simulink model "Model_double_control"  (R2019b)
settings: Solver=FixedStepAuto  StartTime=0.0  StopTime=0.1  RelTol=1e-3
values from neighbouring files (symbols this model uses):
  c = 14.86e-12    (= 1.486e-11)    [Q_fac.m]
  frequency = 13.56e6    (= 13560000)    [Q_fac.m]
  k_mrc = 1/q    [Q_fac.m]
  r = 50    [Q_fac.m]
libraries: simulink x10, nesl_utility x9, ee_lib x7, fl_lib x7, dspstat3 x4, powerlib_meascontrol x4
settings Model: Creator=Kia  LastModifiedBy=Kia

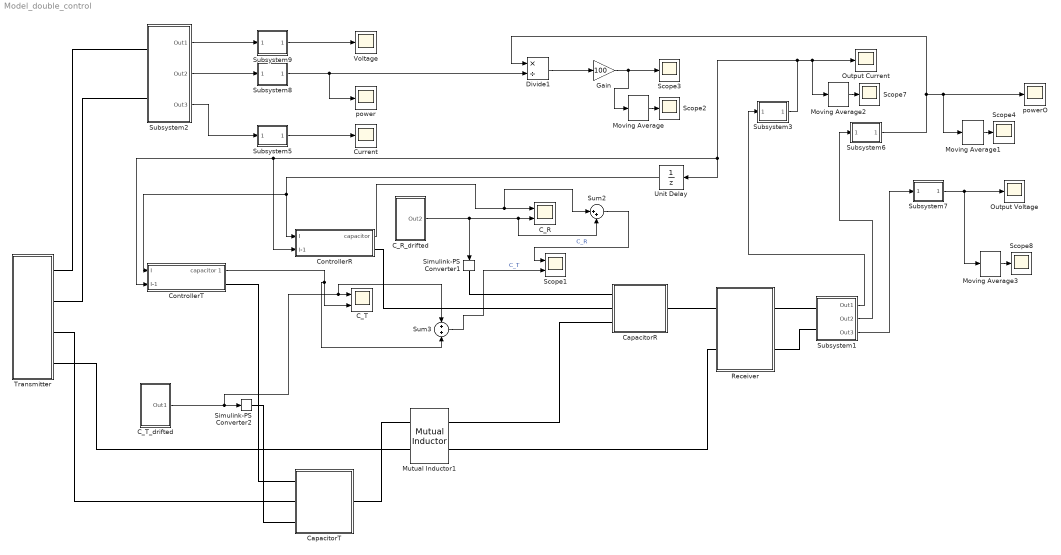
== system Model_double_control ==
  C_R : Scope  NumInputPorts=2
  C_R_drifted : Subsystem
  C_T : Scope  NumInputPorts=2
  C_T_drifted : Subsystem
  CapacitorR : Subsystem
  CapacitorT : Subsystem
  ControllerR : Subsystem
  ControllerT : Subsystem
  Current : Scope
  Divide1 : Product  Inputs=*/
  Gain : Gain  Gain=100
  Moving Average{,1..3} (4 alike) : dspstat3/Moving Average  Method=Sliding window  ForgettingFactorPort=off  SpecifyWindowLength=on  WindowLength=10  ForgettingFactor=0.9  SimulateUsing=Code generation
  Mutual Inductor1 : fl_lib/Electrical/Electrical Elements/Mutual Inductor  L1=l H  L2=l H  k=k_mrc  i1_specify=off  i1_priority=High  i1=0 A  i1_nominal_specify=off  i1_nominal_unit=A  i1_nominal_value=1  i2_specify=off  i2_priority=High  i2=0 A  i2_nominal_specify=off  i2_nominal_unit=A  i2_nominal_value=1  v1_specify=off  v1_priority=None  v1=0 V  v1_nominal_specify=off  v1_nominal_unit=V  v1_nominal_value=1  v2_specify=off  v2_priority=None  v2=0 V  v2_nominal_specify=off  v2_nominal_unit=V  v2_nominal_value=1
      settings: SourceProductName=Simscape  SourceProductBaseCode=SS  InternalSimscapePortConfiguration="{\"Bottom\":[],\"Left\":[{\"id\":\"p1\",\"label\":\"1+\",\"type\":\"foundation.electrical.electrical\"},{\"id\":\"n1\",\"label\":\"1-\",\"type\":\"foundation.electrical.electrical\"}],\"Right\":[{\"id\":\"p2\",\"label\":\"2+\",\"type\":\"foundation.electrical.electrical\"},{\"id\":\"n2\",\"label\":\"2-\",\"type\":\"foundation.electrical.electrical\"}],\"Top\":[]}"
  Output Current : Scope
  Output Voltage : Scope
  Receiver : Subsystem
  Scope1 : Scope  NumInputPorts=2
  Scope{2..4,7..8} (5 alike) : Scope
  Simulink-PS Converter1 : nesl_utility/Simulink-PS Converter  PhysicalDomain=network_engine_domain  SubClassName=ps_input  LeftPortType=input  RightPortType=output  PseudoPeriodic=off  Frequencies=[]  NoiseDistribution=none  NoiseParameters=[]  Unit=1  AffineConversion=off  FilteringAndDerivatives=provide  SimscapeFilterOrder=1  InputFilterTimeConstant=0.001  UdotUserProvided=0
  Simulink-PS Converter2 : nesl_utility/Simulink-PS Converter  PhysicalDomain=network_engine_domain  SubClassName=ps_input  LeftPortType=input  RightPortType=output  PseudoPeriodic=off  Frequencies=[]  NoiseDistribution=none  NoiseParameters=[]  Unit=1  AffineConversion=off  FilteringAndDerivatives=provide  SimscapeFilterOrder=1  InputFilterTimeConstant=0.001  UdotUserProvided=0
  Subsystem1 : Subsystem
  Subsystem2 : Subsystem
  Subsystem3 : Subsystem
  Subsystem5 : Subsystem
  Subsystem6 : Subsystem
  Subsystem7 : Subsystem
  Subsystem8 : Subsystem
  Subsystem9 : Subsystem
  Sum2 : Sum  Inputs=|++
  Sum3 : Sum  Inputs=+|+
  Transmitter : Subsystem
  Unit Delay : UnitDelay  SampleTime=2e-5  HasFrameUpgradeWarning=on
  Voltage : Scope
  power : Scope
  powerO : Scope
  wires:
  Subsystem1/3(Out3) -> Subsystem7/1(In1)
  Subsystem2/3(Out3) -> Subsystem5/1(In1)
  Subsystem1/2(Out2) -> Subsystem6/1(In1)
  Subsystem2/2(Out2) -> Subsystem8/1(In1)
  Subsystem2/1(Out1) -> Subsystem9/1(In1)
  Subsystem1/1(Out1) -> Subsystem3/1(In1)
  ControllerR/1("capacitor ") -> Sum2/1, C_R/1
  Subsystem3/1(Out1) -> Moving Average2/1, Output Current/1, Unit Delay/1, ControllerR/2(I-1), ControllerT/2(I-1)
  Subsystem6/1(Out1) -> Moving Average1/1, powerO/1, Divide1/1
  Divide1/1 -> Gain/1
  C_R_drifted/1(Out2) -> Sum2/2, C_R/2, Simulink-PS Converter1/1
  C_T_drifted/1(Out1) -> Sum3/1, C_T/1, Simulink-PS Converter2/1
  Sum2/1 -> Scope1/1  "C_R"
  Sum3/1 -> Scope1/2  "C_T"
  Unit Delay/1 -> ControllerT/1(I), ControllerR/1(I)
  Subsystem7/1(Out1) -> Moving Average3/1, Output Voltage/1
  Subsystem8/1(Out1) -> power/1, Divide1/2
  Subsystem5/1(Out1) -> Current/1
  Subsystem9/1(Out1) -> Voltage/1
  Gain/1 -> Moving Average/1, Scope3/1
  Moving Average/1 -> Scope2/1
  Moving Average1/1 -> Scope4/1
  Moving Average2/1 -> Scope7/1
  Moving Average3/1 -> Scope8/1
  ControllerT/1(capacitor 1) -> C_T/2, Sum3/2
  connections:
  Receiver/RConn2 -- Subsystem1/LConn2
  Transmitter/RConn3 -- CapacitorT/LConn2
  Transmitter/RConn2 -- Subsystem2/LConn2
  Simulink-PS Converter1/RConn1 -- CapacitorR/LConn1
  Receiver/RConn1 -- Subsystem1/LConn1
  Transmitter/RConn1 -- Subsystem2/LConn1
  Mutual Inductor1/LConn2 -- Transmitter/RConn4
  Mutual Inductor1/RConn2 -- Receiver/LConn2
  Receiver/LConn1 -- CapacitorR/RConn1
  CapacitorR/LConn3 -- Mutual Inductor1/RConn1
  ControllerR/RConn1 -- CapacitorR/LConn2
  CapacitorT/RConn1 -- Mutual Inductor1/LConn1
  Simulink-PS Converter2/RConn1 -- CapacitorT/LConn3
  ControllerT/RConn1 -- CapacitorT/LConn1

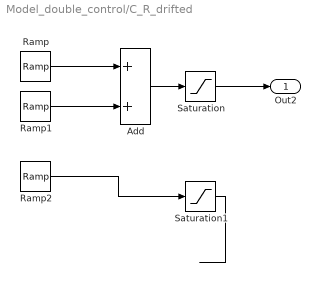
== system Model_double_control/C_R_drifted ==
  Add : Sum
  Ramp : simulink/Sources/Ramp  slope=(0.05*c)*1/2e-4  start=0.015  InitialOutput=0.5*c
  Ramp1 : simulink/Sources/Ramp  slope=-(0.05*c)*2/2e-4  start=0.019  InitialOutput=0
  Ramp2 : simulink/Sources/Ramp  slope=(0.05*c)*1/10e-3  start=0.03  InitialOutput=0.5*c
  Saturation : Saturate  UpperLimit=0.55*c  LowerLimit=c/2
  Saturation1 : Saturate  UpperLimit=0.55*c  LowerLimit=c/2
  Out2 : Outport
  wires:
  Ramp/1 -> Add/1
  Ramp1/1 -> Add/2
  Add/1 -> Saturation/1
  Saturation/1 -> Out2/1
  Saturation1/1 -> ?
  Ramp2/1 -> Saturation1/1

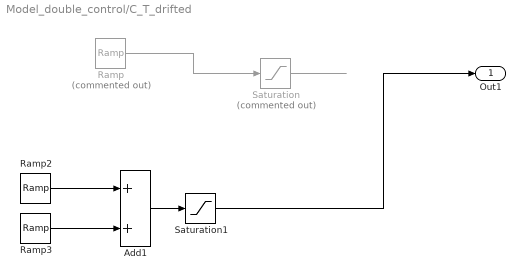
== system Model_double_control/C_T_drifted ==
  Add1 : Sum
  Ramp : simulink/Sources/Ramp  Commented=on  slope=(0.05*c)*1/10e-3  start=1e-4  InitialOutput=0.5*c
  Ramp2 : simulink/Sources/Ramp  slope=(0.05*c)*1/2e-4  start=1e-4  InitialOutput=0.5*c
  Ramp3 : simulink/Sources/Ramp  slope=-(0.05*c)*2/2e-4  start=0.004  InitialOutput=0
  Saturation : Saturate  Commented=on  UpperLimit=0.55*c  LowerLimit=c/2
  Saturation1 : Saturate  UpperLimit=0.55*c  LowerLimit=c/2
  Out1 : Outport
  wires:
  Ramp/1 -> Saturation/1
  Saturation/1 -> ?
  Ramp3/1 -> Add1/2
  Add1/1 -> Saturation1/1
  Ramp2/1 -> Add1/1
  Saturation1/1 -> Out1/1

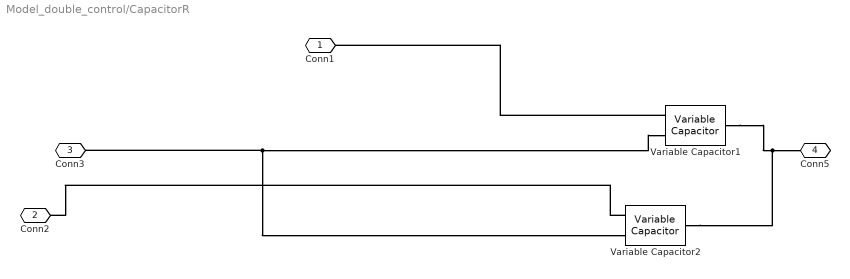
== system Model_double_control/CapacitorR ==
  Variable Capacitor1 : ee_lib/Passive/Variable Capacitor  prm=2  Cmin=1e-20 F  r=0 Ohm  v0=0 V  q0=0 C
      settings: SourceProductName=Simscape Electrical  SourceProductBaseCode=PS  InternalSimscapePortConfiguration="{\"Bottom\":[],\"Left\":[{\"id\":\"C\",\"label\":\"C\",\"type\":\"input\"},{\"id\":\"p\",\"label\":\"+\",\"type\":\"foundation.electrical.electrical\"}],\"Right\":[{\"id\":\"n\",\"label\":\"-\",\"type\":\"foundation.electrical.electrical\"}],\"Top\":[]}"
  Variable Capacitor2 : ee_lib/Passive/Variable Capacitor  prm=2  Cmin=1e-20 F  r=0 Ohm  v0=0 V  q0=0 C
      settings: SourceProductName=Simscape Electrical  SourceProductBaseCode=PS  InternalSimscapePortConfiguration="{\"Bottom\":[],\"Left\":[{\"id\":\"C\",\"label\":\"C\",\"type\":\"input\"},{\"id\":\"p\",\"label\":\"+\",\"type\":\"foundation.electrical.electrical\"}],\"Right\":[{\"id\":\"n\",\"label\":\"-\",\"type\":\"foundation.electrical.electrical\"}],\"Top\":[]}"
  Conn1 : PMIOPort  Side=Left
  Conn2 : PMIOPort  Port=2  Side=Left
  Conn3 : PMIOPort  Port=3  Side=Left
  Conn5 : PMIOPort  Port=4  Side=Right
  connections:
  Variable Capacitor1/LConn1 -- Conn1/RConn1
  Variable Capacitor2/LConn1 -- Conn2/RConn1
  Variable Capacitor1/RConn1 -- Variable Capacitor2/RConn1 -- Conn5/RConn1
  Conn3/RConn1 -- Variable Capacitor2/LConn2 -- Variable Capacitor1/LConn2

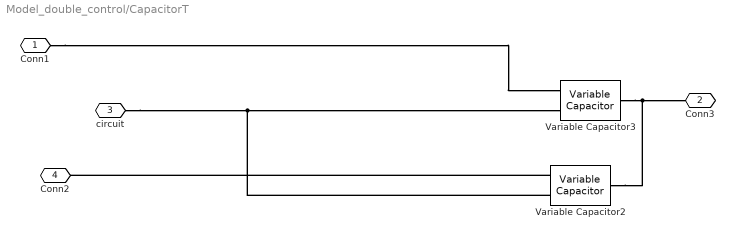
== system Model_double_control/CapacitorT ==
  Variable Capacitor2 : ee_lib/Passive/Variable Capacitor  prm=2  Cmin=1e-20 F  r=0 Ohm  v0=0 V  q0=0 C
      settings: SourceProductName=Simscape Electrical  SourceProductBaseCode=PS  InternalSimscapePortConfiguration="{\"Bottom\":[],\"Left\":[{\"id\":\"C\",\"label\":\"C\",\"type\":\"input\"},{\"id\":\"p\",\"label\":\"+\",\"type\":\"foundation.electrical.electrical\"}],\"Right\":[{\"id\":\"n\",\"label\":\"-\",\"type\":\"foundation.electrical.electrical\"}],\"Top\":[]}"
  Variable Capacitor3 : ee_lib/Passive/Variable Capacitor  prm=2  Cmin=1e-20 F  r=0 Ohm  v0=0 V  q0=0 C
      settings: SourceProductName=Simscape Electrical  SourceProductBaseCode=PS  InternalSimscapePortConfiguration="{\"Bottom\":[],\"Left\":[{\"id\":\"C\",\"label\":\"C\",\"type\":\"input\"},{\"id\":\"p\",\"label\":\"+\",\"type\":\"foundation.electrical.electrical\"}],\"Right\":[{\"id\":\"n\",\"label\":\"-\",\"type\":\"foundation.electrical.electrical\"}],\"Top\":[]}"
  Conn1 : PMIOPort  Side=Left
  Conn3 : PMIOPort  Port=2  Side=Right
  circuit : PMIOPort  Port=3  Side=Left
  Conn2 : PMIOPort  Port=4  Side=Left
  connections:
  Variable Capacitor3/RConn1 -- Variable Capacitor2/RConn1 -- Conn3/RConn1
  circuit/RConn1 -- Variable Capacitor3/LConn2 -- Variable Capacitor2/LConn2
  Variable Capacitor2/LConn1 -- Conn2/RConn1
  Conn1/RConn1 -- Variable Capacitor3/LConn1

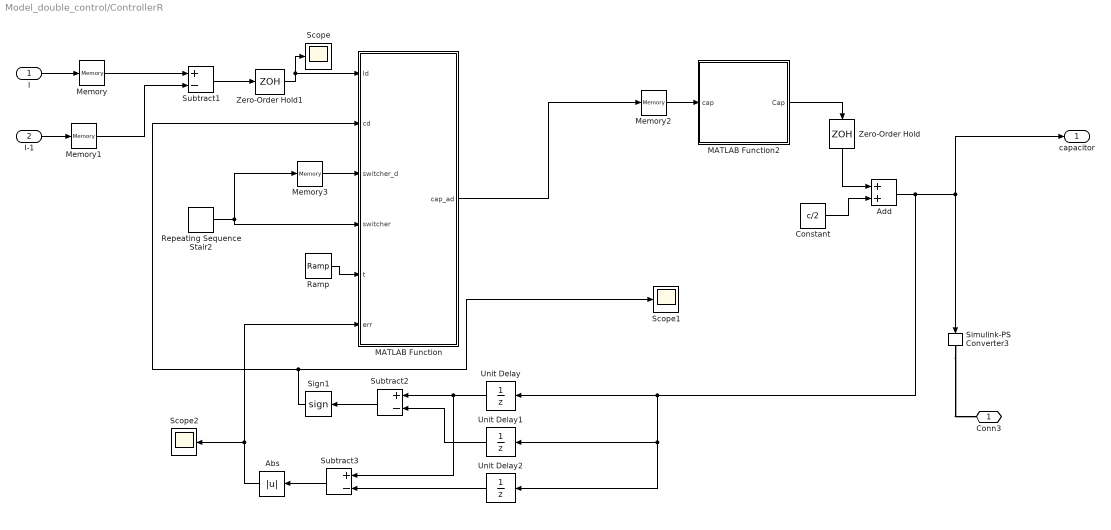
== system Model_double_control/ControllerR ==
  I : Inport
  I-1 : Inport  Port=2
  Abs : Abs
  Add : Sum
  Constant : Constant  Value=c/2  SampleTime=1e-8
  MATLAB Function : MATLAB Function  TreatAsAtomicUnit=on
  MATLAB Function2 : MATLAB Function  TreatAsAtomicUnit=on
  Memory{,1..3} (4 alike) : Memory
  Ramp : simulink/Sources/Ramp  slope=1  start=0  InitialOutput=0
  Repeating Sequence Stair2 : simulink/Sources/Repeating Sequence Stair  OutValues=[0 1 2 3 4 5 6 7 8 0 0 0 0 0 0 0 0 0 0].'  tsamp=2e-5  OutMin=[]  OutMax=[]  OutDataTypeStr=double  OutputDataTypeScalingMode=double  OutDataType=fixdt(0,8)  ConRadixGroup=Best Precision: Vector-wise  OutScaling=2^-12
  Scope : Scope
  Scope1 : Scope
  Scope2 : Scope
  Sign1 : Signum
  Simulink-PS Converter3 : nesl_utility/Simulink-PS Converter  PhysicalDomain=network_engine_domain  SubClassName=ps_input  LeftPortType=input  RightPortType=output  PseudoPeriodic=off  Frequencies=[]  NoiseDistribution=none  NoiseParameters=[]  Unit=1  AffineConversion=off  FilteringAndDerivatives=provide  SimscapeFilterOrder=1  InputFilterTimeConstant=0.001  UdotUserProvided=0
  Subtract1 : Sum  Inputs=+-
  Subtract2 : Sum  Inputs=+-
  Subtract3 : Sum  Inputs=+-
  Unit Delay : UnitDelay  SampleTime=2e-5  HasFrameUpgradeWarning=on
  Unit Delay1 : UnitDelay  SampleTime=4e-5  HasFrameUpgradeWarning=on
  Unit Delay2 : UnitDelay  SampleTime=6e-5  HasFrameUpgradeWarning=on
  Zero-Order Hold : ZeroOrderHold  SampleTime=2e-5
  Zero-Order Hold1 : ZeroOrderHold  SampleTime=2e-5
  Conn3 : PMIOPort  Side=Right
  "capacitor " : Outport
  wires:
  Ramp/1 -> MATLAB Function/5(t)
  Constant/1 -> Add/2
  Unit Delay/1 -> Subtract3/1, Subtract2/1
  Unit Delay1/1 -> Subtract2/2
  Subtract2/1 -> Sign1/1
  Sign1/1 -> Scope1/1, MATLAB Function/2(cd)
  I/1 -> Memory/1
  I-1/1 -> Memory1/1
  Subtract1/1 -> Zero-Order Hold1/1
  Memory/1 -> Subtract1/1
  Memory1/1 -> Subtract1/2
  Add/1 -> Simulink-PS Converter3/1, "capacitor "/1, Unit Delay2/1, Unit Delay1/1, Unit Delay/1
  Memory2/1 -> MATLAB Function2/1(cap)
  MATLAB Function2/1(Cap) -> Zero-Order Hold/1
  Zero-Order Hold/1 -> Add/1
  Zero-Order Hold1/1 -> Scope/1, MATLAB Function/1(Id)
  Unit Delay2/1 -> Subtract3/2
  Subtract3/1 -> Abs/1
  Abs/1 -> Scope2/1, MATLAB Function/6(err)
  Repeating Sequence Stair2/1 -> Memory3/1, MATLAB Function/4(switcher)
  Memory3/1 -> MATLAB Function/3(switcher_d)
  MATLAB Function/1(cap_ad) -> Memory2/1
  connections:
  Simulink-PS Converter3/RConn1 -- Conn3/RConn1

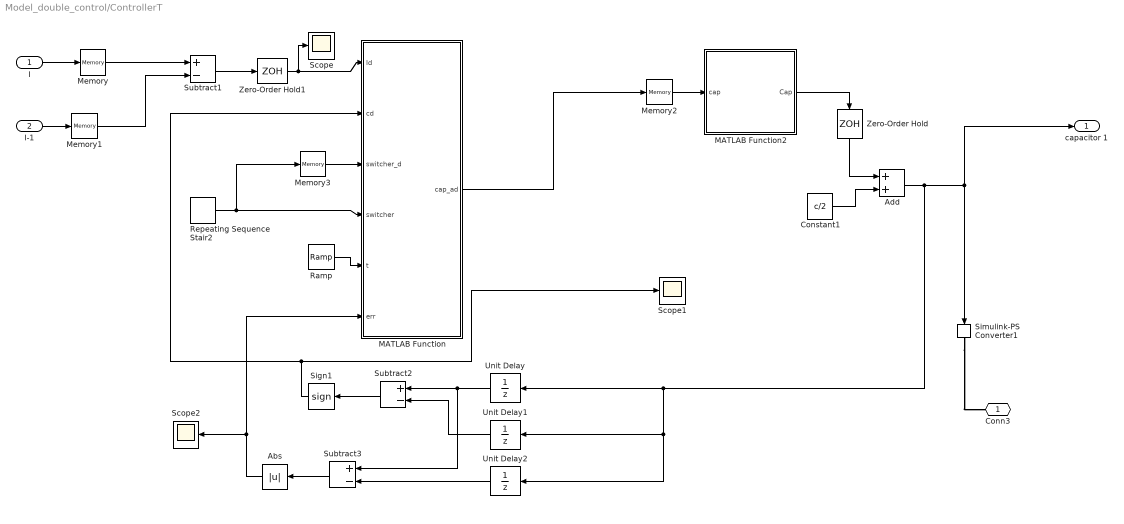
== system Model_double_control/ControllerT ==
  I : Inport
  I-1 : Inport  Port=2
  Abs : Abs
  Add : Sum
  Constant1 : Constant  Value=c/2  SampleTime=1e-8
  MATLAB Function : MATLAB Function  TreatAsAtomicUnit=on
  MATLAB Function2 : MATLAB Function  TreatAsAtomicUnit=on
  Memory{,1..3} (4 alike) : Memory
  Ramp : simulink/Sources/Ramp  slope=1  start=0  InitialOutput=0
  Repeating Sequence Stair2 : simulink/Sources/Repeating Sequence Stair  OutValues=[0 0 0 0 0 0 0 0 0 0 0 1 2 3 4 5 6 7 8].'  tsamp=2e-5  OutMin=[]  OutMax=[]  OutDataTypeStr=double  OutputDataTypeScalingMode=double  OutDataType=fixdt(0,8)  ConRadixGroup=Best Precision: Vector-wise  OutScaling=2^-12
  Scope : Scope
  Scope1 : Scope
  Scope2 : Scope
  Sign1 : Signum
  Simulink-PS Converter1 : nesl_utility/Simulink-PS Converter  PhysicalDomain=network_engine_domain  SubClassName=ps_input  LeftPortType=input  RightPortType=output  PseudoPeriodic=off  Frequencies=[]  NoiseDistribution=none  NoiseParameters=[]  Unit=1  AffineConversion=off  FilteringAndDerivatives=provide  SimscapeFilterOrder=1  InputFilterTimeConstant=0.001  UdotUserProvided=0
  Subtract1 : Sum  Inputs=+-
  Subtract2 : Sum  Inputs=+-
  Subtract3 : Sum  Inputs=+-
  Unit Delay : UnitDelay  SampleTime=2e-5  HasFrameUpgradeWarning=on
  Unit Delay1 : UnitDelay  SampleTime=4e-5  HasFrameUpgradeWarning=on
  Unit Delay2 : UnitDelay  SampleTime=6e-5  HasFrameUpgradeWarning=on
  Zero-Order Hold : ZeroOrderHold  SampleTime=2e-5
  Zero-Order Hold1 : ZeroOrderHold  SampleTime=2e-5
  Conn3 : PMIOPort  Side=Right
  capacitor 1 : Outport
  wires:
  Zero-Order Hold1/1 -> Scope/1, MATLAB Function/1(Id)
  Zero-Order Hold/1 -> Add/1
  MATLAB Function/1(cap_ad) -> Memory2/1
  Abs/1 -> Scope2/1, MATLAB Function/6(err)
  Memory/1 -> Subtract1/1
  Subtract3/1 -> Abs/1
  Unit Delay1/1 -> Subtract2/2
  Unit Delay2/1 -> Subtract3/2
  Memory3/1 -> MATLAB Function/3(switcher_d)
  Unit Delay/1 -> Subtract3/1, Subtract2/1
  Subtract1/1 -> Zero-Order Hold1/1
  Repeating Sequence Stair2/1 -> Memory3/1, MATLAB Function/4(switcher)
  Add/1 -> Simulink-PS Converter1/1, capacitor 1/1, Unit Delay2/1, Unit Delay1/1, Unit Delay/1
  Subtract2/1 -> Sign1/1
  Ramp/1 -> MATLAB Function/5(t)
  Memory1/1 -> Subtract1/2
  I-1/1 -> Memory1/1
  Constant1/1 -> Add/2
  MATLAB Function2/1(Cap) -> Zero-Order Hold/1
  I/1 -> Memory/1
  Sign1/1 -> Scope1/1, MATLAB Function/2(cd)
  Memory2/1 -> MATLAB Function2/1(cap)
  connections:
  Simulink-PS Converter1/RConn1 -- Conn3/RConn1

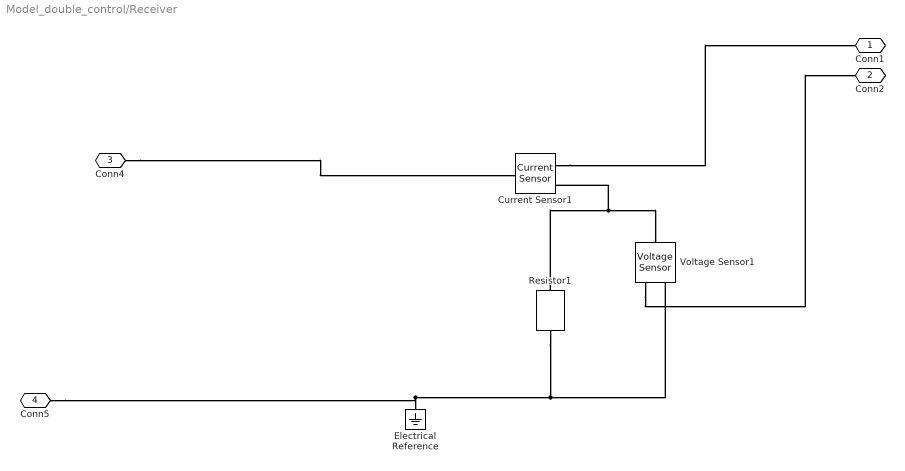
== system Model_double_control/Receiver ==
  Current Sensor1 : fl_lib/Electrical/Electrical Sensors/Current Sensor
  Electrical Reference : fl_lib/Electrical/Electrical Elements/Electrical Reference
  Resistor1 : ee_lib/Passive/Resistor  R=r Ohm  R_tol=1e-20  enable_R_tol=0  tol_distribution=1  nSigma=4  enable_operating_limits=0  operating_limit_action=2  max_working_voltage=100 V  power_rating=1 W  enable_faults=0  fault_action=1  R_faulted=inf Ohm  enable_temporal_fault=0  t_fault=1 s  enable_behavioral_fault=0  max_permissible_current=1 A  t_fail_on_current=1 s  noise_mode=0  sample_time=1e-3 s  repeatability=1  auto_seed=2821191750  user_seed=0  Tdevice=25 degC  alpha=3.93e-3 1/K  Tmeas=25 degC  thermal_mass=100 J/K  power_derating_T1=70 degC  power_derating_T2=155 degC  operating_temperature_range_vec=[-50, 150] degC  temperature_specify=off  temperature_priority=High  temperature=298.15 K  temperature_nominal_specify=off  temperature_nominal_unit=K  temperature_nominal_value=1
      settings: SourceProductName=Simscape Electrical
  Voltage Sensor1 : fl_lib/Electrical/Electrical Sensors/Voltage Sensor
  Conn1 : PMIOPort  Side=Right
  Conn2 : PMIOPort  Port=2  Side=Right
  Conn4 : PMIOPort  Port=3  Side=Left
  Conn5 : PMIOPort  Port=4  Side=Left
  connections:
  Voltage Sensor1/RConn2 -- Electrical Reference/LConn1 -- Conn5/RConn1 -- Resistor1/RConn1
  Current Sensor1/RConn2 -- Resistor1/LConn1 -- Voltage Sensor1/LConn1
  Current Sensor1/RConn1 -- Conn1/RConn1
  Voltage Sensor1/RConn1 -- Conn2/RConn1
  Conn4/RConn1 -- Current Sensor1/LConn1

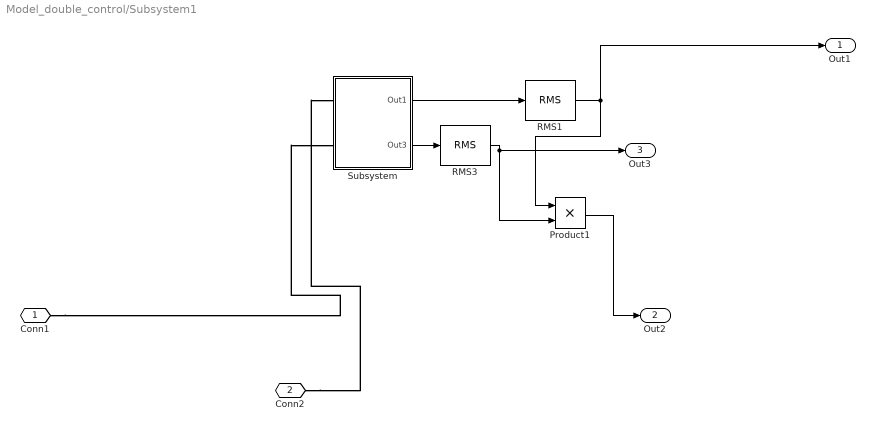
== system Model_double_control/Subsystem1 ==
  Product1 : Product
  RMS1 : powerlib_meascontrol/Measurements/RMS  TrueRMS=on  Freq=frequency  RMSInit=0  Ts=1e-8
      settings: SourceProductName=Simscape Electrical
  RMS3 : powerlib_meascontrol/Measurements/RMS  TrueRMS=on  Freq=frequency  RMSInit=0  Ts=1e-8
      settings: SourceProductName=Simscape Electrical
  Subsystem : Subsystem
  Conn1 : PMIOPort  Side=Left
  Conn2 : PMIOPort  Port=2  Side=Left
  Out1 : Outport
  Out2 : Outport  Port=2
  Out3 : Outport  Port=3
  wires:
  Product1/1 -> Out2/1
  RMS1/1 -> Out1/1, Product1/1
  Subsystem/1(Out1) -> RMS1/1
  RMS3/1 -> Out3/1, Product1/2
  Subsystem/2(Out3) -> RMS3/1
  connections:
  Conn2/RConn1 -- Subsystem/LConn1
  Conn1/RConn1 -- Subsystem/LConn2

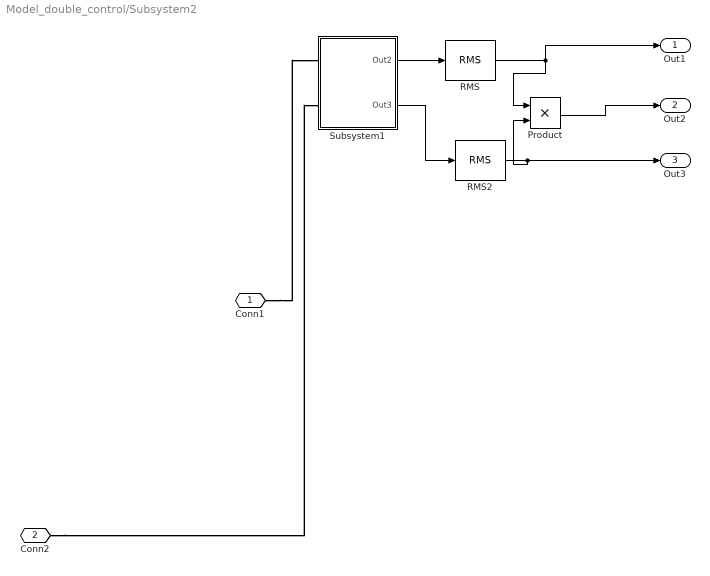
== system Model_double_control/Subsystem2 ==
  Product : Product
  RMS : powerlib_meascontrol/Measurements/RMS  TrueRMS=on  Freq=frequency  RMSInit=0  Ts=1e-8
      settings: SourceProductName=Simscape Electrical
  RMS2 : powerlib_meascontrol/Measurements/RMS  TrueRMS=on  Freq=frequency  RMSInit=0  Ts=1e-8
      settings: SourceProductName=Simscape Electrical
  Subsystem1 : Subsystem
  Conn1 : PMIOPort  Side=Left
  Conn2 : PMIOPort  Port=2  Side=Left
  Out1 : Outport
  Out2 : Outport  Port=2
  Out3 : Outport  Port=3
  wires:
  RMS/1 -> Out1/1, Product/1
  Subsystem1/2(Out3) -> RMS2/1
  RMS2/1 -> Out3/1, Product/2
  Product/1 -> Out2/1
  Subsystem1/1(Out2) -> RMS/1
  connections:
  Conn2/RConn1 -- Subsystem1/LConn2
  Conn1/RConn1 -- Subsystem1/LConn1

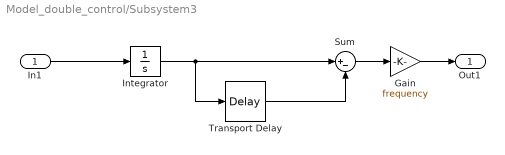
== system Model_double_control/Subsystem3 ==
  In1 : Inport
  Gain : Gain  Gain=frequency
  Integrator : Integrator
  Sum : Sum  Inputs=|+-
  Transport Delay : TransportDelay  DelayTime=1/frequency
  Out1 : Outport
  wires:
  Gain/1 -> Out1/1
  Transport Delay/1 -> Sum/2
  Integrator/1 -> Transport Delay/1, Sum/1
  In1/1 -> Integrator/1
  Sum/1 -> Gain/1

== system Model_double_control/Subsystem5 ==
  In1 : Inport
  Gain : Gain  Gain=frequency
  Integrator : Integrator
  Sum : Sum  Inputs=|+-
  Transport Delay : TransportDelay  DelayTime=1/frequency
  Out1 : Outport
  wires:
  Gain/1 -> Out1/1
  Transport Delay/1 -> Sum/2
  Integrator/1 -> Transport Delay/1, Sum/1
  In1/1 -> Integrator/1
  Sum/1 -> Gain/1

== system Model_double_control/Subsystem6 ==
  In1 : Inport
  Gain : Gain  Gain=frequency
  Integrator : Integrator
  Sum : Sum  Inputs=|+-
  Transport Delay : TransportDelay  DelayTime=1/frequency
  Out1 : Outport
  wires:
  Gain/1 -> Out1/1
  Transport Delay/1 -> Sum/2
  Integrator/1 -> Transport Delay/1, Sum/1
  In1/1 -> Integrator/1
  Sum/1 -> Gain/1

== system Model_double_control/Subsystem7 ==
  In1 : Inport
  Gain : Gain  Gain=frequency
  Integrator : Integrator
  Sum : Sum  Inputs=|+-
  Transport Delay : TransportDelay  DelayTime=1/frequency
  Out1 : Outport
  wires:
  Gain/1 -> Out1/1
  Transport Delay/1 -> Sum/2
  Integrator/1 -> Transport Delay/1, Sum/1
  In1/1 -> Integrator/1
  Sum/1 -> Gain/1

== system Model_double_control/Subsystem8 ==
  In1 : Inport
  Gain : Gain  Gain=frequency
  Integrator : Integrator
  Sum : Sum  Inputs=|+-
  Transport Delay : TransportDelay  DelayTime=1/frequency
  Out1 : Outport
  wires:
  Gain/1 -> Out1/1
  Transport Delay/1 -> Sum/2
  Integrator/1 -> Transport Delay/1, Sum/1
  In1/1 -> Integrator/1
  Sum/1 -> Gain/1

== system Model_double_control/Subsystem9 ==
  In1 : Inport
  Gain : Gain  Gain=frequency
  Integrator : Integrator
  Sum : Sum  Inputs=|+-
  Transport Delay : TransportDelay  DelayTime=1/frequency
  Out1 : Outport
  wires:
  Gain/1 -> Out1/1
  Transport Delay/1 -> Sum/2
  Integrator/1 -> Transport Delay/1, Sum/1
  In1/1 -> Integrator/1
  Sum/1 -> Gain/1

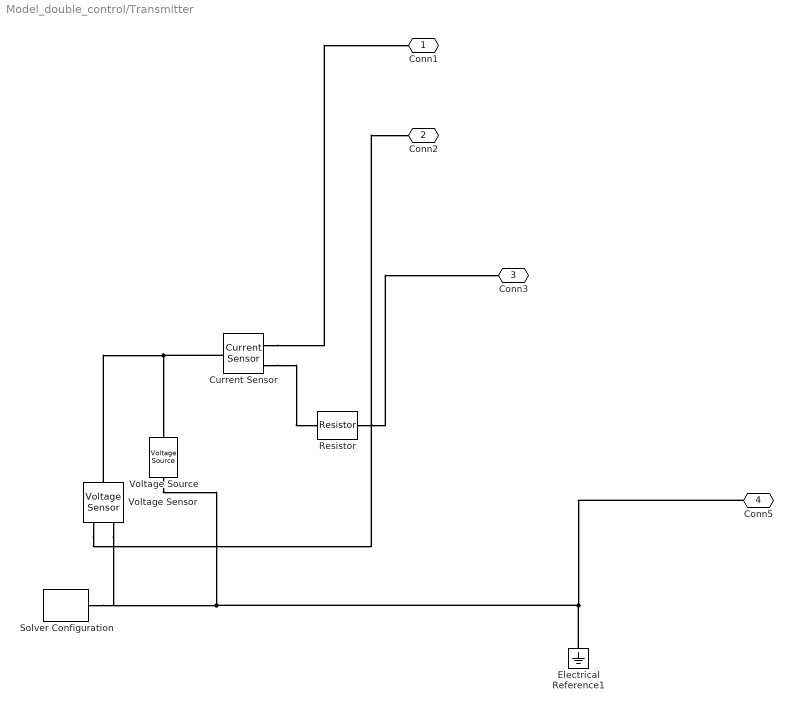
== system Model_double_control/Transmitter ==
  Current Sensor : fl_lib/Electrical/Electrical Sensors/Current Sensor
  Electrical Reference1 : fl_lib/Electrical/Electrical Elements/Electrical Reference
  Resistor : ee_lib/Passive/Resistor  R=r Ohm  R_tol=1e-20  enable_R_tol=0  tol_distribution=1  nSigma=4  enable_operating_limits=0  operating_limit_action=2  max_working_voltage=100 V  power_rating=1 W  enable_faults=0  fault_action=1  R_faulted=inf Ohm  enable_temporal_fault=0  t_fault=1 s  enable_behavioral_fault=0  max_permissible_current=1 A  t_fail_on_current=1 s  noise_mode=0  sample_time=1e-3 s  repeatability=1  auto_seed=2697125040  user_seed=0  Tdevice=25 degC  alpha=3.93e-3 1/K  Tmeas=25 degC  thermal_mass=100 J/K  power_derating_T1=70 degC  power_derating_T2=155 degC  operating_temperature_range_vec=[-50, 150] degC  temperature_specify=off  temperature_priority=High  temperature=298.15 K  temperature_nominal_specify=off  temperature_nominal_unit=K  temperature_nominal_value=1
      settings: SourceProductName=Simscape Electrical
  Solver Configuration : nesl_utility/Solver Configuration  PhysicalDomain=network_engine_domain  SubClassName=solver  LeftPortType=input  RightPortType=generic  Tones=[]  Harmonics=[]  SimulateNoise=off  Profile=off  UseLocalSampling=off  EnableSwitchedLinearOptims=on  FrequencyDomain=off  UseCCode=off  RelTol=0.001  AbsTol=1e-06  MinStep=1e-09  ToWorkspace=off  RevertToSquareIcSolve=off  NumHomotopyIterations=100  PhasorMode=off  PhasorModeNumHarmonics=1  DoDC=off  ResidualTolerance=1e-15  UseLocalSolver=off  LocalSolverChoice=NE_BACKWARD_EULER_ADVANCER  LocalSolverSampleTime=0.001  DoFixedCost=off  MaxNonlinIter=3  MaxModeIter=2  LinearAlgebra=auto  EquationFormulation=NE_TIME_EF  DelaysMemoryBudget=1024  AutomaticFiltering=off  FilteringTimeConstant=0.0001  PartitionStorageMethod=AS_NEEDED  PartitionMemoryBudget=1024  PartitionMethod=ROBUST
  Voltage Sensor : fl_lib/Electrical/Electrical Sensors/Voltage Sensor
  Voltage Source : ee_lib/Sources/Voltage Source  dc_voltage=0 V  ac_voltage=1 V  ac_shift=0 deg  ac_frequency=frequency Hz  noise_mode=0  PSD=0 V^2/Hz  repeatability=1  auto_seed=1254062075  user_seed=0  sample_time=1e-3 s  i_specify=off  i_priority=None  i=0 A  i_nominal_specify=off  i_nominal_unit=A  i_nominal_value=1  v_specify=off  v_priority=None  v=0 V  v_nominal_specify=off  v_nominal_unit=V  v_nominal_value=1
      settings: SourceProductName=Simscape Electrical
  Conn1 : PMIOPort  Side=Right
  Conn2 : PMIOPort  Port=2  Side=Right
  Conn3 : PMIOPort  Port=3  Side=Right
  Conn5 : PMIOPort  Port=4  Side=Right
  connections:
  Electrical Reference1/LConn1 -- Conn5/RConn1 -- Solver Configuration/RConn1 -- Voltage Sensor/RConn2 -- Voltage Source/RConn1
  Resistor/RConn1 -- Conn3/RConn1
  Current Sensor/RConn2 -- Resistor/LConn1
  Voltage Sensor/RConn1 -- Conn2/RConn1
  Current Sensor/RConn1 -- Conn1/RConn1
  Current Sensor/LConn1 -- Voltage Sensor/LConn1 -- Voltage Source/LConn1

== system Model_double_control/Subsystem1/Subsystem ==
  PS-Simulink Converter : nesl_utility/PS-Simulink Converter  PhysicalDomain=network_engine_domain  SubClassName=ps_output  LeftPortType=input  RightPortType=output  PseudoPeriodic=off  Frequencies=[]  Unit=inherit  AffineConversion=off
  PS-Simulink Converter1 : nesl_utility/PS-Simulink Converter  PhysicalDomain=network_engine_domain  SubClassName=ps_output  LeftPortType=input  RightPortType=output  PseudoPeriodic=off  Frequencies=[]  Unit=inherit  AffineConversion=off
  Conn1 : PMIOPort  Side=Left
  Conn2 : PMIOPort  Port=2  Side=Left
  Out1 : Outport
  Out3 : Outport  Port=2
  wires:
  PS-Simulink Converter/1 -> Out1/1
  PS-Simulink Converter1/1 -> Out3/1
  connections:
  PS-Simulink Converter1/LConn1 -- Conn1/RConn1
  Conn2/RConn1 -- PS-Simulink Converter/LConn1

== system Model_double_control/Subsystem2/Subsystem1 ==
  PS-Simulink Converter2 : nesl_utility/PS-Simulink Converter  PhysicalDomain=network_engine_domain  SubClassName=ps_output  LeftPortType=input  RightPortType=output  PseudoPeriodic=off  Frequencies=[]  Unit=inherit  AffineConversion=off
  PS-Simulink Converter3 : nesl_utility/PS-Simulink Converter  PhysicalDomain=network_engine_domain  SubClassName=ps_output  LeftPortType=input  RightPortType=output  PseudoPeriodic=off  Frequencies=[]  Unit=inherit  AffineConversion=off
  Conn1 : PMIOPort  Side=Left
  Conn2 : PMIOPort  Port=2  Side=Left
  Out2 : Outport
  Out3 : Outport  Port=2
  wires:
  PS-Simulink Converter2/1 -> Out2/1
  PS-Simulink Converter3/1 -> Out3/1
  connections:
  Conn2/RConn1 -- PS-Simulink Converter2/LConn1
  PS-Simulink Converter3/LConn1 -- Conn1/RConn1

== matlab function Model_double_control/ControllerR/MATLAB Function ==
  settings: updateMethod=DISCRETE
  data: cap_ad output; Id input; cd input; switcher_d input; switcher input; t input; err input
function cap_ad = adjust_capacitor(Id, cd, switcher_d, switcher, t, err)

% step = 5e-17;
step = 2e-17;
eps=0;
min_I=1e-8;
if t<1.1e-4
    cap_ad=0;
elseif (switcher==1)
    cap_ad= step/5;
elseif switcher>=2 && Id>=min_I && err>1e-17
    if switcher_d==1
        cap_ad = -sign(cd)*step+eps;
    elseif switcher_d>=2
        cap_ad = -sign(cd)*((0.9)^(switcher_d-1))*step+eps;
    else
        cap_ad = -sign(cd)*step+eps;
    end
elseif switcher>=2 && Id<-min_I && err>1e-17
    if switcher_d==1
        cap_ad = +sign(cd)*step+eps;
    elseif switcher_d>=2
        cap_ad = +sign(cd)*((0.9)^(switcher_d-1))*step+eps;
    else
        cap_ad = +sign(cd)*step+eps;
    end
else 
    cap_ad = eps;
end
end

== matlab function Model_double_control/ControllerT/MATLAB Function ==
  data: cap_ad output; Id input; cd input; switcher_d input; switcher input; t input; err input
function cap_ad = adjust_capacitor(Id, cd, switcher_d, switcher, t, err)

% step = 5e-17;
step = 2e-17;
eps=0;
min_I=1e-8;
if t<1.1e-4
    cap_ad=0;
elseif (switcher==1)
    cap_ad= step/5;
elseif switcher>=2 && Id>=min_I && err>1e-17
    if switcher_d==1
        cap_ad = -sign(cd)*step+eps;
    elseif switcher_d>=2
        cap_ad = -sign(cd)*((0.9)^(switcher_d-1))*step+eps;
    else
        cap_ad = -sign(cd)*step+eps;
    end
elseif switcher>=2 && Id<-min_I && err>1e-17
    if switcher_d==1
        cap_ad = +sign(cd)*step+eps;
    elseif switcher_d>=2
        cap_ad = +sign(cd)*((0.9)^(switcher_d-1))*step+eps;
    else
        cap_ad = +sign(cd)*step+eps;
    end
else 
    cap_ad = eps;
end
end

== matlab function Model_double_control/ControllerT/MATLAB Function2 ==
  settings: updateMethod=DISCRETE
  data: cap input; Cap output
function Cap = adjust_capacitor(cap)
persistent C
if isempty(C)
    C = 0;
end
C=C+cap
Cap=C;
end

== matlab function Model_double_control/ControllerR/MATLAB Function2 ==
  settings: updateMethod=DISCRETE
  data: cap input; Cap output
function Cap = adjust_capacitor(cap)
persistent C
if isempty(C)
    C = 0;
end
C=C+cap
Cap=C;
end
